simulink model "p_model_elec_and_mech"  (R2021a)
settings: Solver=ode15s  StartTime=0.0  StopTime=3  FixedStep=0.0001  RelTol=0.01
InitFcn:
  | p_init;
values from neighbouring files (symbols this model uses):
  a = 0    [p_init.m]
  b = 1/1.34e6    (= 7.46268656716e-07)    [p_init.m]
  B_r = t_0/w_0    (= 3.31437084591e-07)    [p_init.m]
  enc_res = 0.875 * pi/180    (= 0.015271630955)    [p_init.m]
  J_a = J_a/(gear_ratio^2)    (= 1.4693877551e-07)    [p_init.m]    (also in p_init_wrist.m = J_a/(gear_ratio_w^2))
  J_r = 0.939 * 1e-7    (= 9.39e-08)    [p_init.m]
  K_b = 1/(327*2*pi/60)    (= 0.0292027418517)    [p_init.m]
  K_m = 29.2 / 1000    (= 0.0292)    [p_init.m]
  K_p = 4.72e6/1.34e6    (= 3.5223880597)    [p_init.m]
  L_term = 1.61 / 1000    (= 0.00161)    [p_init.m]
  R_term = 37.1    [p_init.m]
  v_max_amp = +V_nom    (= 24)    [p_init.m]
  v_min_amp = -V_nom    (= -24)    [p_init.m]
libraries: pid_lib x1
settings Model: Creator=Konstantin  LastModifiedBy=kossio
settings SolverCC: ZeroCrossControl=DisableAll  AlgebraicLoopSolver=TrustRegion
settings DebuggingCC: SFMachineParentedDataDiag=warning

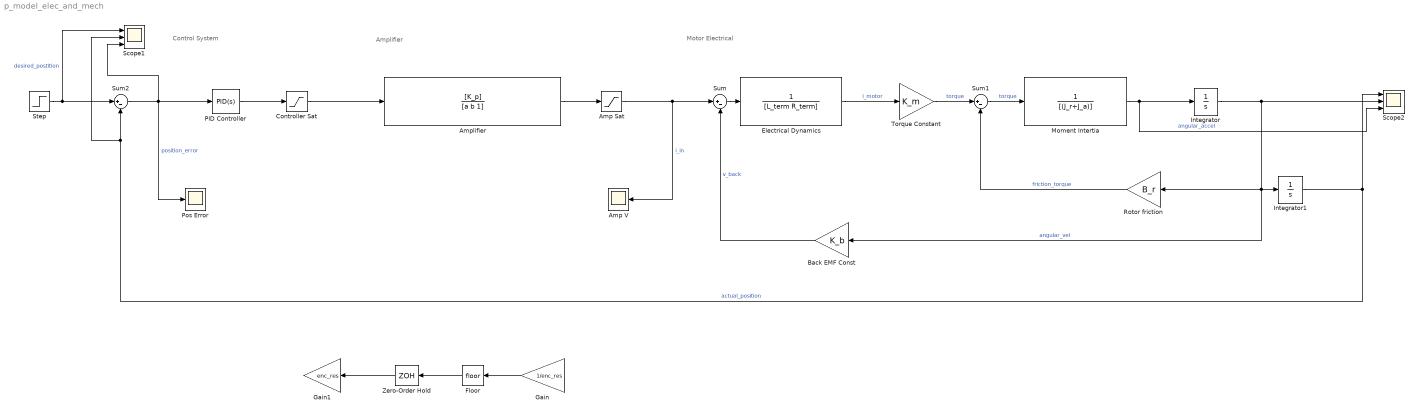
== system p_model_elec_and_mech ==
  note: Control System
  note: Motor Electrical
  note: Amplifier
  Amp Sat : Saturate  UpperLimit=v_max_amp  LowerLimit=v_min_amp
  Amp V : Scope
  Amplifier : TransferFcn  Numerator=[K_p]  Denominator=[a b 1]
  Back EMF Const : Gain  Gain=K_b
  Controller Sat : Saturate  UpperLimit=10  LowerLimit=-10
  Electrical Dynamics : TransferFcn  Denominator=[L_term R_term]
  Floor : Rounding
  Gain : Gain  Gain=1/enc_res
  Gain1 : Gain  Gain=enc_res
  Integrator : Integrator
  Integrator1 : Integrator
  Moment Intertia : TransferFcn  Denominator=[(J_r+J_a)]
  PID Controller : pid_lib/PID Controller  Controller=PID  Form=Parallel  TimeDomain=Continuous-time  UseExternalTs=off  SampleTime=-1  IntegratorMethod=Forward Euler  FilterMethod=Forward Euler  ControllerParametersSource=internal  P=1  I=0  D=0  UseFilter=on  N=100  TunerSelectOption=Transfer Function Based (PID Tuner App)  InitialConditionSource=internal  InitialConditionForIntegrator=0  InitialConditionForFilter=0  DifferentiatorICPrevScaledInput=0  ExternalReset=none  TrackingMode=off  Kt=1  LimitOutput=off  SatLimitsSource=internal  UpperSaturationLimit=inf  LowerSaturationLimit=-inf  LinearizeAsGain=on  AntiWindupMode=none  Kb=1  POutMin=[]  POutMax=[]  IOutMin=[]  IOutMax=[]  DOutMin=[]  DOutMax=[]  NOutMin=[]  NOutMax=[]  SumOutMin=[]  SumOutMax=[]  SaturationOutMin=[]  SaturationOutMax=[]  PParamMin=[]  PParamMax=[]  IParamMin=[]  IParamMax=[]  DParamMin=[]  DParamMax=[]  NParamMin=[]  NParamMax=[]  KbParamMin=[]  KbParamMax=[]  KtParamMin=[]  KtParamMax=[]  KbOutMin=[]  KbOutMax=[]  KtOutMin=[]  KtOutMax=[]  IntegratorOutMin=[]  IntegratorOutMax=[]  FilterOutMin=[]  FilterOutMax=[]  SumI1OutMin=[]  SumI1OutMax=[]  SumI2OutMin=[]  SumI2OutMax=[]  SumI3OutMin=[]  SumI3OutMax=[]  SumI4OutMin=[]  SumI4OutMax=[]  SumDOutMin=[]  SumDOutMax=[]  DifferentiatorOutMin=[]  DifferentiatorOutMax=[]  FilterDiffOutCoefMin=[]  FilterDiffOutCoefMax=[]  ReciprocalOutMin=[]  ReciprocalOutMax=[]  SumDenOutMin=[]  SumDenOutMax=[]  SumNumOutMin=[]  SumNumOutMax=[]  DivideOutMin=[]  DivideOutMax=[]  UdiffTsProdOutMin=[]  UdiffTsProdOutMax=[]  NTsProdOutMin=[]  NTsProdOutMax=[]  UintegralTsProdOutMin=[]  UintegralTsProdOutMax=[]  UngainTsProdOutMin=[]  UngainTsProdOutMax=[]  IntegratorContinuousStateAttributes=''  IntegratorStateMustResolveToSignalObject=off  IntegratorRTWStateStorageClass=Auto  FilterContinuousStateAttributes=''  FilterStateMustResolveToSignalObject=off  FilterRTWStateStorageClass=Auto  ParallelPVariant=InternalParameters  IdealPVariant=Disabled  IVariant=InternalParameters  DVariant=InternalParameters  IntegratorVariant=Continuous  SatVariant=Disabled  AWVariant=Passthrough  PCopyVariant=Disabled  TRVariant=Disabled  FdbkBlocksVariant=Forward  IdealPFdbkVariant=Disabled  SatFdbkVariant=Disabled  DerivativeFilterVariant=ContFilter  NVariant=InternalParameters  NCopyVariant=Disabled  FilterICVariant=InternalICsFilter  IntegratorICVariant=InternalICs  ExternalResetVariant=Disabled  TRSumVariant=Passthrough  SumFdbkVariant=Disabled  SumVariant=Sum_PID  TsampFilterVariant=InternalTs  TsampNgainVariant=Passthrough  TsampIntegralVariant=Passthrough  ExternalSaturationOutDataTypeStr=Inherit: Same as second input
  Pos Error : Scope
  Rotor friction : Gain  Gain=B_r
  Scope1 : Scope  NumInputPorts=3
  Scope2 : Scope  NumInputPorts=3
  Step : Step  Time=0  After=pi/2  SampleTime=0
  Sum : Sum  Inputs=|+-
  Sum1 : Sum  Inputs=|+-
  Sum2 : Sum  Inputs=|+-
  Torque Constant : Gain  Gain=K_m
  Zero-Order Hold : ZeroOrderHold  SampleTime=0.001
  wires:
  Sum/1 -> Electrical Dynamics/1
  Electrical Dynamics/1 -> Torque Constant/1  "i_motor"
  Amp Sat/1 -> Sum/1, Amp V/1  "i_in"
  Controller Sat/1 -> Amplifier/1
  Amplifier/1 -> Amp Sat/1
  Back EMF Const/1 -> Sum/2  "v_back"
  Moment Intertia/1 -> Scope2/3, Integrator/1  "angular_accel"
  Integrator/1 -> Scope2/2, Integrator1/1, Back EMF Const/1, Rotor friction/1  "angular_vel"
  Rotor friction/1 -> Sum1/2  "friction_torque"
  Torque Constant/1 -> Sum1/1  "torque"
  Sum1/1 -> Moment Intertia/1  "torque"
  Sum2/1 -> PID Controller/1, Scope1/3, Pos Error/1  "position_error"
  Step/1 -> Scope1/1, Sum2/1  "desired_postition"
  Integrator1/1 -> Sum2/2, Scope1/2, Scope2/1  "actual_position"
  Zero-Order Hold/1 -> Gain1/1
  Floor/1 -> Zero-Order Hold/1
  Gain/1 -> Floor/1
  PID Controller/1 -> Controller Sat/1
